simulink model "fixpt_ovf"  (R2015b)
settings: Solver=FixedStepDiscrete  StartTime=0.0  StopTime=10  RelTol=1e-3
settings Model: Creator=y_yama  LastModifiedBy=amatsumo
settings DataIOCC: SaveFormat=Array  SignalLoggingSaveFormat=ModelDataLogs  SaveOutput=off  SaveTime=off
settings OptimizationCC: BlockReduction=off  ConditionallyExecuteInputs=off  DefaultParameterBehavior=Inlined  InlineInvariantSignals=on  ExpressionDepthLimit=2147483647  ZeroExternalMemoryAtStartup=off  ZeroInternalMemoryAtStartup=off  InitFltsAndDblsToZero=on  NoFixptDivByZeroProtection=on  EfficientFloat2IntCast=on  OptimizeModelRefInitCode=on  LifeSpan=1
settings DebuggingCC: UnderspecifiedInitializationDetection=Classic  MergeDetectMultiDrivingBlocksExec=none  SolverPrmCheckMsg=warning  InheritedTsInSrcMsg=none  FcnCallInpInsideContextMsg=UseLocalSettings  StateNameClashWarn=warning
settings HardwareCC: ProdBitPerPointer=32  ProdLargestAtomicFloat=None  ProdWordSize=32  ProdHWDeviceType=Generic->32-bit Embedded Processor
settings RTWCC: SystemTargetFile=ert.tlc  GenCodeOnly=on  TemplateMakefile=ert_default_tmf  Description=Real-Time Workshop Embedded Coder (no auto configuration)  GenerateReport=on  IncludeHyperlinkInReport=on  LaunchReport=on
settings CodeAppCC: GenerateComments=off  IgnoreCustomStorageClasses=off  CustomSymbolStrGlobalVar=$N$M  CustomSymbolStrType=$N$R$M  SimulinkBlockComments=off  InternalIdentifier=Classic
settings ERTTargetCC: GenerateSampleERTMain=on  IncludeMdlTerminateFcn=off  SuppressErrorStatus=on  SupportAbsoluteTime=off  SupportNonFinite=off  SupportComplex=off  PurelyIntegerCode=on  InlinedParameterPlacement=NonHierarchical  ERTCustomFileTemplate=example_file_process.tlc
settings ConfigComp: CovModelRefEnable=Off  CovSFcnEnable=off

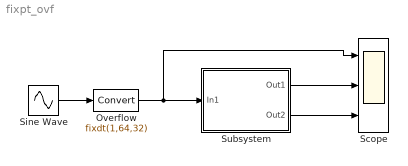
== system fixpt_ovf ==
  Overflow : DataTypeConversion  OutDataTypeStr=fixdt(1,64,32)  RndMeth=Nearest
  Scope : Scope  NumInputPorts=3
  Sine Wave : Sin  Amplitude=4  SampleTime=1/1000
      settings: AttributesFormatString=Amplitude = %<Amplitude>
  Subsystem : Subsystem
  wires:
  Subsystem/1(Out1) -> Scope/2
  Sine Wave/1 -> Overflow/1
  Overflow/1 -> Scope/1, Subsystem/1(In1)
  Subsystem/2(Out2) -> Scope/3

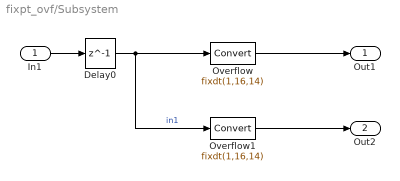
== system fixpt_ovf/Subsystem ==
  In1 : Inport
  Delay0 : Delay  DelayLength=1  InitialCondition=0
  Overflow : DataTypeConversion  OutDataTypeStr=fixdt(1,16,14)  RndMeth=Nearest
      settings: AttributesFormatString=OutDataType: %<OutDataTypeStr>\nSaturation: %<SaturateOnIntegerOverflow>
  Overflow1 : DataTypeConversion  OutDataTypeStr=fixdt(1,16,14)  RndMeth=Nearest  SaturateOnIntegerOverflow=on
      settings: AttributesFormatString=OutDataType: %<OutDataTypeStr>\nSaturation: %<SaturateOnIntegerOverflow>
  Out1 : Outport
  Out2 : Outport  Port=2
  wires:
  Delay0/1 -> Overflow1/1, Overflow/1  "in1"
  In1/1 -> Delay0/1
  Overflow/1 -> Out1/1
  Overflow1/1 -> Out2/1
